simulink model "A3_2"  (R2016b)
settings: Solver=VariableStepAuto  StartTime=0.0  StopTime=28  RelTol=1e-3
settings Model: Creator=jonathankirchman  LastModifiedBy=jonathankirchman

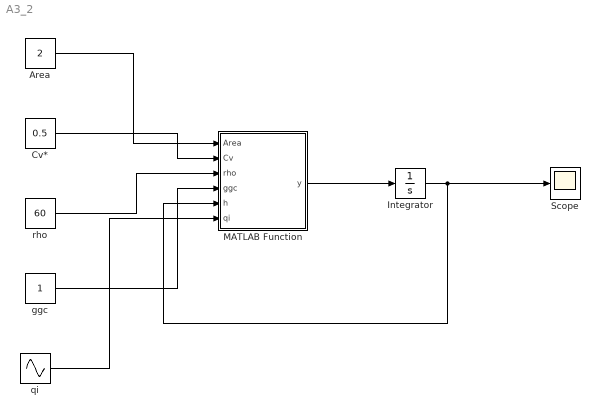
== system A3_2 ==
  Area : Constant  Value=2
  Cv* : Constant  Value=0.5
  Integrator : Integrator  InitialCondition=10
  MATLAB Function : MATLAB Function  TreatAsAtomicUnit=on
  Scope : Scope
  ggc : Constant
  qi : Sin  SampleTime=0
  rho : Constant  Value=60
  wires:
  Area/1 -> MATLAB Function/1(Area)
  Cv*/1 -> MATLAB Function/2(Cv)
  rho/1 -> MATLAB Function/3(rho)
  ggc/1 -> MATLAB Function/4(ggc)
  MATLAB Function/1(y) -> Integrator/1
  Integrator/1 -> MATLAB Function/5(h), Scope/1
  qi/1 -> MATLAB Function/6(qi)

== matlab function A3_2/MATLAB Function ==
  data: Area input; y output; Cv input; rho input; ggc input; h input; qi input
function y = fcn(Area,Cv,rho,ggc,h,qi) 

Cvv = Cv*sqrt(ggc);
y = qi/Area-Cvv*sqrt(h(1))/Area;
